simulink model "identifica_ip02"  (Simulink 9.2)
settings: Solver=ode4  StartTime=0.0  StopTime=3  FixedStep=0.001  RelTol=1e-3  AbsTol=1e-6  EnableMultiTasking=on
values from neighbouring files (symbols this model uses):
  a = 2*qsi*wn    [identifica.m]    (also in magik.mat = 11.7382904175; magik2.mat = 11.7382904175; setup_lab_ip01_2.m = 1)
  b = wn^2 /420    [identifica.m]    (also in magik.mat = 1.43067670553; magik2.mat = 1.43067670553; setup_lab_ip01_2.m = 1)
  K_AMP = 1    [magik.mat]    (also in magik2.mat; setup_lab_ip01_2.m)
  K_EC = 2.27485440932e-05    [magik.mat]    (also in magik2.mat; setup_ip01_2_configuration.m)
  K_EP = 0.00153398078789    [magik.mat]    (also in magik2.mat; setup_ip01_2_configuration.m)
  qsi = log(1/MP)/sqrt(pi^2 + (log(1/MP))^2)    [identifica.m]    (also in magik.mat = 0.239430491122; magik2.mat = 0.239430491122; setup_lab_ip01_2.m = 1)
  VMAX_AMP = 12    [magik.mat]    (also in magik2.mat; setup_ip01_2_configuration.m = 4.16)
  VMAX_DAC = 10    [magik.mat]    (also in magik2.mat; setup_lab_ip01_2.m)
  wn = pi/(tp*sqrt(1-qsi^2))    [identifica.m]    (also in magik.mat = 24.5129397732; magik2.mat = 24.5129397732; setup_lab_ip01_2.m = 1)
  X_LIM_ENABLE = 1    [magik.mat]    (also in magik2.mat; setup_lab_ip01_2.m)
  X_MAX = 0.3    [magik.mat]    (also in magik2.mat; setup_lab_ip01_2.m)
  X_MIN = -0.3    [magik.mat]    (also in magik2.mat; setup_lab_ip01_2.m)
undefined symbols (not defined in the file or in its folder): HIL, qc_get_step_size
libraries: quarc_library x5, simulink_extras x1
CloseFcn:
  | rtwprivate ssgencode ModelCloseRequest q_position_pv_ip02
settings Model: Creator=Mfotoohi  LastModifiedBy=Andre Almeida  ExtModeTrigDuration=50000
settings SolverCC: AutoScaleAbsTol=off  PositivePriorityOrder=on
settings DataIOCC: LimitDataPoints=off
settings OptimizationCC: BooleanDataType=off  OptimizeBlockIOStorage=off  BufferReuse=off  GlobalBufferReuse=off  ExpressionFolding=off  ExpressionDepthLimit=2147483647  LocalBlockOutputs=off  InitFltsAndDblsToZero=on  OptimizeDataStoreBuffers=off  BusAssignmentInplaceUpdate=off
settings DebuggingCC: SaveWithParameterizedLinksMsg=none  SignalResolutionControl=TryResolveAllWithWarning  MultiTaskDSMMsg=warning  MultiTaskCondExecSysMsg=none
settings HardwareCC: TargetHWDeviceType=32-bit Generic
settings RTWCC: SystemTargetFile=quarc_windows.tlc  TemplateMakefile=quarc_default_tmf  Description=Quarc Win32 Target
settings STFCustomTargetCC: TargetFcnLib=ansi_tfl_tmw.mat  TargetPreCompLibLocation=C:\DOCUME~1\ALLUSE~1\DADOSD~1\QUARC\lib\2008b\windows\release  CPPClassGenCompliant=on  SystemTargetFile=quarc_windows.tlc
settings GRTTargetCC: TargetFcnLib=ansi_tfl_tmw.mat  TargetPreCompLibLocation=C:\DOCUME~1\ALLUSE~1\DADOSD~1\QUARC\lib\2008b\windows\release  ParMdlRefBuildCompliant=off  CompOptLevelCompliant=off  ConcurrentExecutionCompliant=off  GeneratePreprocessorConditionals=Use local settings  MatFileLogging=off  UseToolchainInfoCompliant=off  ExtMode=on  ExtModeMexFile=quarc_comm
settings ConfigComp: CovExternalEMLEnable=on

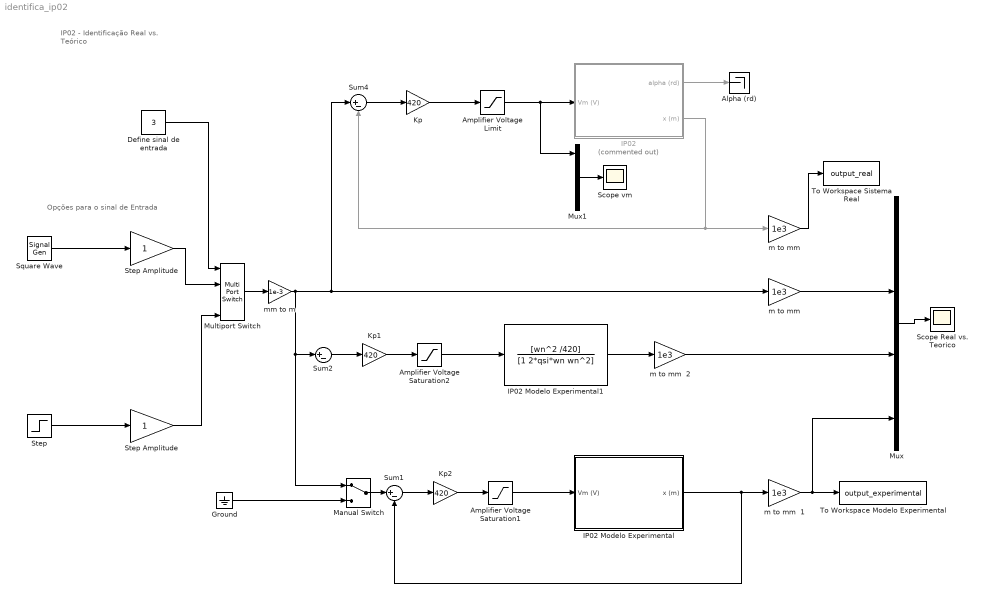
== system identifica_ip02 ==
  note: IP02 - Identificação
      | Real vs. Teórico
  note: Opções para o sinal de Entrada
  Alpha (rd) : Terminator
  Amplifier Voltage Limit : Saturate  UpperLimit=VMAX_AMP  LowerLimit=- VMAX_AMP
  Amplifier Voltage Saturation1 : Saturate  UpperLimit=VMAX_AMP  LowerLimit=- VMAX_AMP
  Amplifier Voltage Saturation2 : Saturate  UpperLimit=VMAX_AMP  LowerLimit=- VMAX_AMP
  Define sinal de entrada : Constant  Value=3
  Ground : Ground
  IP02 : Subsystem  Commented=on
  IP02 Modelo Experimental : Subsystem
  IP02 Modelo Experimental1 : TransferFcn  Numerator=[wn^2 /420]  Denominator=[1 2*qsi*wn wn^2]
  Kp : Gain  Gain=420  SaturateOnIntegerOverflow=on  OutDataTypeStr=Inherit: Same as input  ParamDataTypeStr=Inherit: Same as input
  Kp1 : Gain  Gain=420  SaturateOnIntegerOverflow=on  OutDataTypeStr=Inherit: Same as input  ParamDataTypeStr=Inherit: Same as input
  Kp2 : Gain  Gain=420  SaturateOnIntegerOverflow=on  OutDataTypeStr=Inherit: Same as input  ParamDataTypeStr=Inherit: Same as input
  Manual Switch : ManualSwitch
  Multiport Switch : MultiPortSwitch
  Mux : Mux
  Mux1 : Mux  Inputs=3
  Scope Real vs. Teorico : Scope
  Scope vm : Scope
  Square Wave : SignalGenerator  WaveForm=square  Frequency=0.66
  Step : Step  Time=0  SampleTime=0
  Step Amplitude : Gain  SaturateOnIntegerOverflow=on  OutDataTypeStr=Inherit: Same as input  ParamDataTypeStr=Inherit: Same as input
  "Step Amplitude " : Gain  SaturateOnIntegerOverflow=on  OutDataTypeStr=Inherit: Same as input  ParamDataTypeStr=Inherit: Same as input
  Sum1 : Sum  Inputs=|+-  SaturateOnIntegerOverflow=on  InputSameDT=on  OutDataTypeStr=Inherit: Same as first input
  Sum2 : Sum  Inputs=|+-  SaturateOnIntegerOverflow=on  InputSameDT=on  OutDataTypeStr=Inherit: Same as first input
  Sum4 : Sum  Inputs=|+-  SaturateOnIntegerOverflow=on  InputSameDT=on  OutDataTypeStr=Inherit: Same as first input
  To Workspace Modelo Experimental : ToWorkspace  VariableName=output_experimental  SaveFormat=Structure With Time  SampleTime=-1
  To Workspace Sistema Real : ToWorkspace  VariableName=output_real  SaveFormat=Structure With Time  SampleTime=-1
  m to mm : Gain  Gain=1e3  SaturateOnIntegerOverflow=on  OutDataTypeStr=Inherit: Same as input  ParamDataTypeStr=Inherit: Same as input
  "m to mm " : Gain  Gain=1e3  SaturateOnIntegerOverflow=on  OutDataTypeStr=Inherit: Same as input  ParamDataTypeStr=Inherit: Same as input
  m to mm  1 : Gain  Gain=1e3  SaturateOnIntegerOverflow=on  OutDataTypeStr=Inherit: Same as input  ParamDataTypeStr=Inherit: Same as input
  m to mm  2 : Gain  Gain=1e3  SaturateOnIntegerOverflow=on  OutDataTypeStr=Inherit: Same as input  ParamDataTypeStr=Inherit: Same as input
  mm to m : Gain  Gain=1e-3
  wires:
  IP02/2(x (m)) -> m to mm/1, Sum4/2
  Sum4/1 -> Kp/1
  Mux/1 -> Scope Real vs. Teorico/1
  Amplifier Voltage Limit/1 -> IP02/1(Vm (V)), Mux1/1
  IP02/1(alpha (rd)) -> Alpha (rd)/1
  Step Amplitude/1 -> Multiport Switch/2
  Kp/1 -> Amplifier Voltage Limit/1
  Define sinal de entrada/1 -> Multiport Switch/1
  "Step Amplitude "/1 -> Multiport Switch/4
  Step/1 -> "Step Amplitude "/1
  m to mm/1 -> To Workspace Sistema Real/1
  Square Wave/1 -> Step Amplitude/1
  Multiport Switch/1 -> mm to m/1
  Ground/1 -> Manual Switch/2
  Mux1/1 -> Scope vm/1
  Sum1/1 -> Kp2/1
  IP02 Modelo Experimental/1(x (m)) -> Sum1/2, m to mm  1/1
  Kp2/1 -> Amplifier Voltage Saturation1/1
  Amplifier Voltage Saturation1/1 -> IP02 Modelo Experimental/1(Vm (V))
  m to mm  1/1 -> To Workspace Modelo Experimental/1, Mux/4
  Manual Switch/1 -> Sum1/1
  m to mm  2/1 -> Mux/3
  "m to mm "/1 -> Mux/2
  mm to m/1 -> Sum2/1, Manual Switch/1, Sum4/1, "m to mm "/1
  Sum2/1 -> Kp1/1
  Amplifier Voltage Saturation2/1 -> IP02 Modelo Experimental1/1
  Kp1/1 -> Amplifier Voltage Saturation2/1
  IP02 Modelo Experimental1/1 -> m to mm  2/1

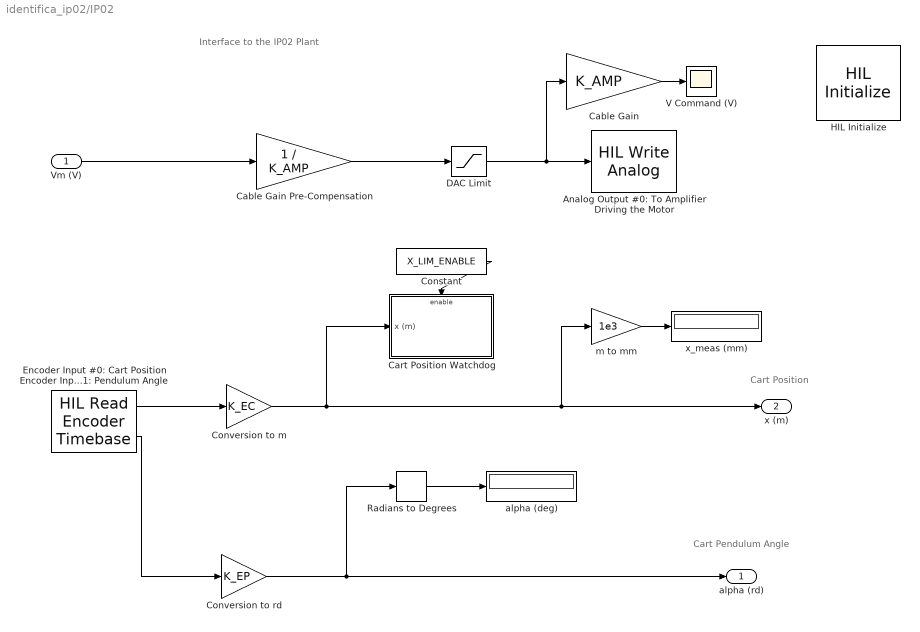
== system identifica_ip02/IP02 ==
  note: Cart Pendulum Angle
  note: Cart Position
  note: Interface to the IP02 Plant
  Vm (V) : Inport
  Analog Output #0: To Amplifier Driving the Motor : quarc_library/Data Acquisition/Generic/Immediate I//O/HIL Write Analog  Tag=unassigned  object_name=HIL-1  channels=0  sample_time=-1  active=on  vector_input=on
  Cable Gain : Gain  Gain=K_AMP  SaturateOnIntegerOverflow=on  OutDataTypeStr=Inherit: Same as input  ParamDataTypeStr=Inherit: Same as input
  Cable Gain Pre-Compensation : Gain  Gain=1 / K_AMP  SaturateOnIntegerOverflow=on  OutDataTypeStr=Inherit: Same as input  ParamDataTypeStr=Inherit: Same as input
  Cart Position Watchdog : Subsystem  TreatAsAtomicUnit=on
  Constant : Constant  Value=X_LIM_ENABLE
  Conversion to m : Gain  Gain=K_EC  SaturateOnIntegerOverflow=on  OutDataTypeStr=Inherit: Same as input  ParamDataTypeStr=Inherit: Same as input
  Conversion to rd : Gain  Gain=K_EP  SaturateOnIntegerOverflow=on  OutDataTypeStr=Inherit: Same as input  ParamDataTypeStr=Inherit: Same as input
  DAC Limit : Saturate  UpperLimit=VMAX_DAC  LowerLimit=- VMAX_DAC
  Encoder Input #0: Cart Position Encoder Input #1: Pendulum Angle : quarc_library/Data Acquisition/Generic/Timebases/HIL Read Encoder Timebase  Tag=unassigned  object_name=HIL-1  clock=0  channels=[0,1]  samples_in_buffer=max(ceil(1/qc_get_step_size), 1)  active=on  vector_output=off  data_type_mode=Inherit via back propagation  data_type=double
  HIL Initialize : quarc_library/Data Acquisition/Generic/Configuration/HIL Initialize  object_name=HIL-1  board_type=q8_usb  board_number=0  board_options=update_rate=normal  exclusive=off  active=off  hardware_clocks=[0:2]  clock_modes=[]  set_clock_params_at_start=off  set_clock_params_at_switch_in=off  analog_input_channels=[0:7]  analog_input_maximums=10  analog_input_minimums=-10  set_analog_input_params_at_start=on  set_analog_input_params_at_switch_in=off  analog_output_channels=[0:7]  analog_output_maximums=10  analog_output_minimums=-10  initial_analog_outputs=[0]  final_analog_outputs=[0]  watchdog_analog_outputs=0  set_analog_output_params_at_start=on  set_analog_output_params_at_switch_in=off  set_analog_outputs_at_start=on  set_analog_outputs_at_switch_in=off  set_analog_outputs_at_terminate=on  set_analog_outputs_at_switch_out=off  set_analog_outputs_on_watchdog=off  digital_input_channels=[]  digital_output_channels=[0:7]  digital_output_configuration=[]  initial_digital_outputs=[0]  final_digital_outputs=[0]  watchdog_digital_outputs=[0]  set_digital_output_params_at_start=off  set_digital_output_params_at_switch_in=off  set_digital_outputs_at_start=on  set_digital_outputs_at_switch_in=off  set_digital_outputs_at_terminate=on  set_digital_outputs_at_switch_out=off  set_digital_outputs_on_watchdog=off  encoder_channels=[0:7]  quadrature=[4]  encoder_filter_frequency=[]  initial_encoder_counts=[0]  set_encoder_params_at_start=on  set_encoder_params_at_switch_in=off  set_encoder_counts_at_start=on  set_encoder_counts_at_switch_in=off  pwm_channels=[0:7]  pwm_modes=0  pwm_frequency=99.532799999999995e6/4095  pwm_configuration=[0]  pwm_alignment=[0]  pwm_polarity=[1]  pwm_leading_deadband=[0]  pwm_trailing_deadband=[0]  initial_pwm_outputs=[0]  final_pwm_outputs=[0]  watchdog_pwm_outputs=[0]  set_pwm_params_at_start=on  set_pwm_params_at_switch_in=off  set_pwm_outputs_at_start=on  set_pwm_outputs_at_switch_in=off  set_pwm_outputs_at_terminate=on  set_pwm_outputs_at_switch_out=off  set_pwm_outputs_on_watchdog=off  other_output_channels=[]  initial_other_outputs=[]  final_other_outputs=[]  watchdog_other_outputs=[]  set_other_outputs_at_start=off  set_other_outputs_at_switch_in=off  set_other_outputs_at_terminate=off  set_other_outputs_at_switch_out=off  set_other_outputs_on_watchdog=off
  Radians to Degrees : simulink_extras/Transformations/Radians to Degrees
  V Command (V) : Scope
  alpha (deg) : Display
      settings: Decimation=100
  m to mm : Gain  Gain=1e3  SaturateOnIntegerOverflow=on  OutDataTypeStr=Inherit: Same as input  ParamDataTypeStr=Inherit: Same as input
  x_meas (mm) : Display
      settings: Decimation=100
  alpha (rd) : Outport  InitialOutput=0
  x (m) : Outport  Port=2  InitialOutput=0
  wires:
  Encoder Input #0: Cart Position Encoder Input #1: Pendulum Angle/1 -> Conversion to m/1
  Conversion to m/1 -> Cart Position Watchdog/1(x (m)), x (m)/1, m to mm/1
  Cable Gain Pre-Compensation/1 -> DAC Limit/1
  m to mm/1 -> x_meas (mm)/1
  Encoder Input #0: Cart Position Encoder Input #1: Pendulum Angle/2 -> Conversion to rd/1
  Radians to Degrees/1 -> alpha (deg)/1
  Conversion to rd/1 -> Radians to Degrees/1, alpha (rd)/1
  Constant/1 -> Cart Position Watchdog/Enable
  DAC Limit/1 -> Analog Output #0: To Amplifier Driving the Motor/1, Cable Gain/1
  Vm (V)/1 -> Cable Gain Pre-Compensation/1
  Cable Gain/1 -> V Command (V)/1

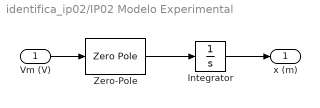
== system identifica_ip02/IP02 Modelo Experimental ==
  Vm (V) : Inport
  Integrator : Integrator
  Zero-Pole : ZeroPole  Zeros=[]  Poles=[-a]  Gain=[b]
  x (m) : Outport
  wires:
  Zero-Pole/1 -> Integrator/1
  Vm (V)/1 -> Zero-Pole/1
  Integrator/1 -> x (m)/1

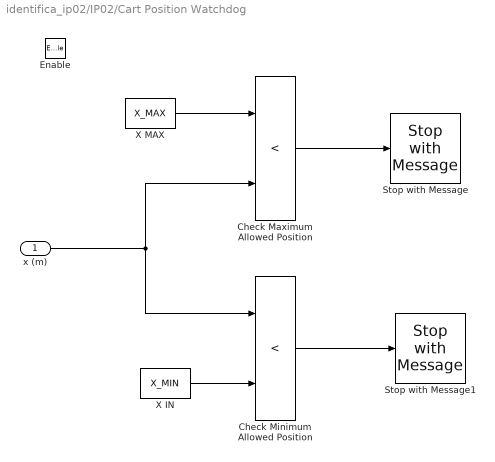
== system identifica_ip02/IP02/Cart Position Watchdog ==
  x (m) : Inport
  Enable : EnablePort
  Check Maximum Allowed Position : RelationalOperator  Operator=<  RndMeth=Nearest  InputSameDT=on
  Check Minimum Allowed Position : RelationalOperator  Operator=<  RndMeth=Nearest  InputSameDT=on
  Stop with Message : quarc_library/Sinks/Error Handling/Stop with Message  SystemSampleTime=-1  message_type=Fixed error message  message_icon=Error  message=Maximum Limit Reached.
  Stop with Message1 : quarc_library/Sinks/Error Handling/Stop with Message  SystemSampleTime=-1  message_type=Fixed error message  message_icon=Error  message=Minimum Limit Reached.
  X IN : Constant  Value=X_MIN
  X MAX : Constant  Value=X_MAX
  wires:
  Check Maximum Allowed Position/1 -> Stop with Message/1
  x (m)/1 -> Check Minimum Allowed Position/1, Check Maximum Allowed Position/2
  X IN/1 -> Check Minimum Allowed Position/2
  Check Minimum Allowed Position/1 -> Stop with Message1/1
  X MAX/1 -> Check Maximum Allowed Position/1
